simulink model "pend_non_linear"  (R2018b)
settings: Solver=ode15s  StartTime=0.0  StopTime=10  MaxStep=0.2  RelTol=1e-6
values from neighbouring files (symbols this model uses):
  Jm = 3.1e-7    (= 3.1e-07)    [main.m]
  Jp = 1774.274e-6    (= 0.001774274)    [main.m]
  Kf = 7.44e-3    (= 0.00744)    [main.m]
  La = 35e-6    (= 3.5e-05)    [main.m]
  lb = 141.451e-3    (= 0.141451)    [main.m]
  M = 879.5e-3    (= 0.8795)    [main.m]
  m = 135.4e-3    (= 0.1354)    [main.m]
  r = 0.01    [main.m]
  Ra = 3.92    [main.m]
  Rg = (13.55+11.04)/4    (= 6.1475)    [main.m]
  rt = 0.01    [main.m]
libraries: simulink x1
settings Model: Creator=Tulio  LastModifiedBy=Giorgio

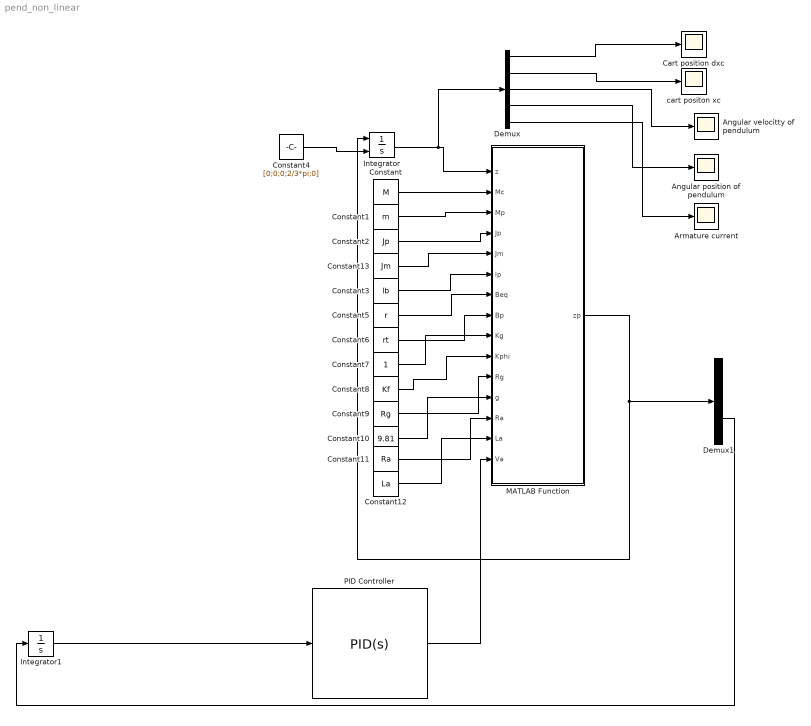
== system pend_non_linear ==
  Angular position of pendulum : Scope
  "Angular velocitty of pendulum " : Scope
  Armature current : Scope
  Cart position dxc : Scope
  Constant : Constant  Value=M
  Constant1 : Constant  Value=m
  Constant10 : Constant  Value=9.81
  Constant11 : Constant  Value=Ra
  Constant12 : Constant  Value=La
  Constant13 : Constant  Value=Jm
  Constant2 : Constant  Value=Jp
  Constant3 : Constant  Value=lb
  Constant4 : Constant  Value=[0;0;0;2/3*pi;0]
  Constant5 : Constant  Value=r
  Constant6 : Constant  Value=rt
  Constant7 : Constant
  Constant8 : Constant  Value=Kf
  Constant9 : Constant  Value=Rg
  Demux : Demux  Outputs=5
  Demux1 : Demux  Outputs=5
  Integrator : Integrator  InitialConditionSource=external
  Integrator1 : Integrator
  MATLAB Function : MATLAB Function  TreatAsAtomicUnit=on
  PID Controller : simulink/Continuous/PID Controller  Controller=PID  Form=Parallel  TimeDomain=Continuous-time  SampleTime=-1  IntegratorMethod=Forward Euler  FilterMethod=Forward Euler  ControllerParametersSource=internal  P=1  I=1  D=1  UseFilter=on  N=100  TunerSelectOption=Transfer Function Based (PID Tuner App)  InitialConditionSource=internal  InitialConditionForIntegrator=0  InitialConditionForFilter=0  DifferentiatorICPrevScaledInput=0  ExternalReset=none  TrackingMode=off  Kt=1  LimitOutput=off  UpperSaturationLimit=inf  LowerSaturationLimit=-inf  LinearizeAsGain=on  AntiWindupMode=none  Kb=1  POutMin=[]  POutMax=[]  IOutMin=[]  IOutMax=[]  DOutMin=[]  DOutMax=[]  NOutMin=[]  NOutMax=[]  SumOutMin=[]  SumOutMax=[]  SaturationOutMin=[]  SaturationOutMax=[]  PParamMin=[]  PParamMax=[]  IParamMin=[]  IParamMax=[]  DParamMin=[]  DParamMax=[]  NParamMin=[]  NParamMax=[]  KbParamMin=[]  KbParamMax=[]  KtParamMin=[]  KtParamMax=[]  KbOutMin=[]  KbOutMax=[]  KtOutMin=[]  KtOutMax=[]  IntegratorOutMin=[]  IntegratorOutMax=[]  FilterOutMin=[]  FilterOutMax=[]  SumI1OutMin=[]  SumI1OutMax=[]  SumI2OutMin=[]  SumI2OutMax=[]  SumI3OutMin=[]  SumI3OutMax=[]  SumI4OutMin=[]  SumI4OutMax=[]  SumDOutMin=[]  SumDOutMax=[]  DifferentiatorOutMin=[]  DifferentiatorOutMax=[]  FilterDiffOutCoefMin=[]  FilterDiffOutCoefMax=[]  ReciprocalOutMin=[]  ReciprocalOutMax=[]  SumDenOutMin=[]  SumDenOutMax=[]  SumNumOutMin=[]  SumNumOutMax=[]  DivideOutMin=[]  DivideOutMax=[]  IntegratorContinuousStateAttributes=''  IntegratorStateMustResolveToSignalObject=off  IntegratorRTWStateStorageClass=Auto  FilterContinuousStateAttributes=''  FilterStateMustResolveToSignalObject=off  FilterRTWStateStorageClass=Auto  ParallelPVariant=InternalParameters  IdealPVariant=Disabled  IVariant=InternalParameters  DVariant=InternalParameters  IntegratorVariant=Continuous  SatVariant=Disabled  AWVariant=Passthrough  PCopyVariant=Disabled  TRVariant=Disabled  FdbkBlocksVariant=Forward  IdealPFdbkVariant=Disabled  SatFdbkVariant=Disabled  DerivativeFilterVariant=ContFilter  NVariant=InternalParameters  NCopyVariant=Disabled  FilterICVariant=InternalICsFilter  IntegratorICVariant=InternalICs  ExternalResetVariant=Disabled  TRSumVariant=Passthrough  SumFdbkVariant=Disabled  SumVariant=Sum_PID
  cart positon xc : Scope
  wires:
  MATLAB Function/1(zp) -> Integrator/1, Demux1/1
  Integrator/1 -> Demux/1, MATLAB Function/1(z)
  Constant/1 -> MATLAB Function/2(Mc)
  Constant1/1 -> MATLAB Function/3(Mp)
  Constant2/1 -> MATLAB Function/4(Jp)
  Constant3/1 -> MATLAB Function/6(lp)
  Constant4/1 -> Integrator/2
  Constant5/1 -> MATLAB Function/7(Beq)
  Constant6/1 -> MATLAB Function/8(Bp)
  Constant7/1 -> MATLAB Function/9(Kg)
  Constant8/1 -> MATLAB Function/10(Kphi)
  Constant9/1 -> MATLAB Function/11(Rg)
  Constant10/1 -> MATLAB Function/12(g)
  Constant11/1 -> MATLAB Function/13(Ra)
  Constant12/1 -> MATLAB Function/14(La)
  Constant13/1 -> MATLAB Function/5(Jm)
  Demux/2 -> cart positon xc/1
  Demux/4 -> Angular position of pendulum/1
  Demux/3 -> "Angular velocitty of pendulum "/1
  Demux/5 -> Armature current/1
  PID Controller/1 -> MATLAB Function/15(Va)
  Demux/1 -> Cart position dxc/1
  Integrator1/1 -> PID Controller/1
  Demux1/4 -> Integrator1/1

== matlab function pend_non_linear/MATLAB Function ==
  data: z input; zp output; Mc input; Mp input; Jp input; Jm input; lp input; Beq input; Bp input; Kg input; Kphi input; Rg input; g input; Ra input; La input; Va input
function zp = fcn(z,Mc,Mp,Jp,Jm,lp,Beq,Bp,Kg,Kphi,Rg,g,Ra,La,Va)
% z = [xcp xc thetap theta Ia]
xcp = z(1); xc = z(2); thetap = z(3); theta = z(4); Ia = z(5);
AA = [Mc+Mp+Jm*(Kg/Rg)^2,0,-Mp*lp*cos(theta),0,0;
      0,1,0,0,0;
      -Mp*lp*cos(theta),0,Jp+Mp*lp^2,0,0;
      0,0,0,1,0;
      0,0,0,0,1];
F = [-Mp*lp*sin(theta)*thetap^2 - Beq*xcp - Kg*Kphi/Rg*Ia;
     xcp;
     -Bp*thetap - Mp*lp*g*sin(theta);
     thetap;
     -Ra/La*Ia - Kg*Kphi/Rg/La*xcp;
    ];
B = [0;0;0;0;1/La];

zp = inv(AA)*F+B*Va;

end
